simulink model "sim_sub_sys_mechanical"  (R2015a)
settings: Solver=ode45  StartTime=0.0  StopTime=10.0  RelTol=1e-3
undefined symbols (not defined in the file or in its folder): beq, Jeq, Tleq
settings Model: Creator=mauric  LastModifiedBy=mauric

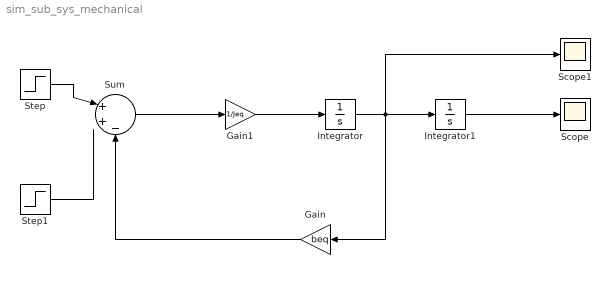
== system sim_sub_sys_mechanical ==
  Gain : Gain  Gain=beq
  Gain1 : Gain  Gain=1/Jeq
  Integrator : Integrator
  Integrator1 : Integrator
  Scope : Scope
  Scope1 : Scope
  Step : Step  After=3  SampleTime=0
  Step1 : Step  After=Tleq  SampleTime=0
  Sum : Sum  Inputs=|++-
  wires:
  Step/1 -> Sum/1
  Step1/1 -> ?
  Gain/1 -> Sum/3
  Sum/1 -> Gain1/1
  Gain1/1 -> Integrator/1
  Integrator/1 -> Gain/1, Scope1/1, Integrator1/1
  Integrator1/1 -> Scope/1
